simulink model "VehicleModel_Embedded"  (R2022a)
settings: Solver=FixedStepAuto  StartTime=0.0  StopTime=10.0  FixedStep=0.2  RelTol=1e-3
model workspace: external: MAT-File InitialValueFile.mat (data not in the file)
values from neighbouring files (symbols this model uses):
  DRIVER_EYES_OFF = Simulink.Parameter    [InitialValueFile.m]
  DRIVER_EYES_ON = Simulink.Parameter    [InitialValueFile.m]
  DRIVER_READINESS_HIGH = Simulink.Parameter    [InitialValueFile.m]
  DRIVER_READINESS_MEDIUM = Simulink.Parameter    [InitialValueFile.m]
  DRIVER_SEATED_ON = Simulink.Parameter    [InitialValueFile.m]
libraries: simulink x6
settings Model: Creator=HP  LastModifiedBy=HP
settings OptimizationCC: DefaultParameterBehavior=Inlined  EnhancedBackFolding=on  PassReuseOutputArgsAs=Individual arguments  ZeroExternalMemoryAtStartup=off  ZeroInternalMemoryAtStartup=off  OptimizeBlockOrder=speed  DifferentSizesBufferReuse=on  OptimizationCustomize=off  EfficientTunableParamExpr=on
settings DebuggingCC: ParameterTunabilityLossMsg=error
settings SFSimCC: MATLABDynamicMemAlloc=off
settings RTWCC: SystemTargetFile=ert.tlc  GenCodeOnly=on  TemplateMakefile=ert_default_tmf
settings CodeAppCC: ForceParamTrailComments=on  IgnoreCustomStorageClasses=off  OperatorAnnotations=on  SimulinkDataObjDesc=on  SFDataObjDesc=on  InsertBlockDesc=on
settings ERTTargetCC: TargetLangStandard=C99 (ISO)  GenerateSampleERTMain=on  InlinedParameterPlacement=NonHierarchical  ERTCustomFileTemplate=example_file_process.tlc

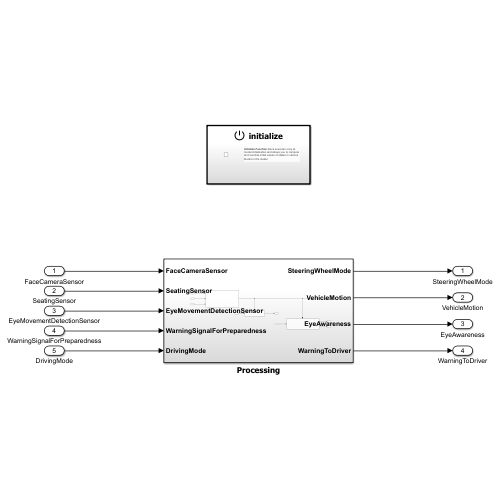
[thumbnail: Simulink's stored preview of the top-level diagram]
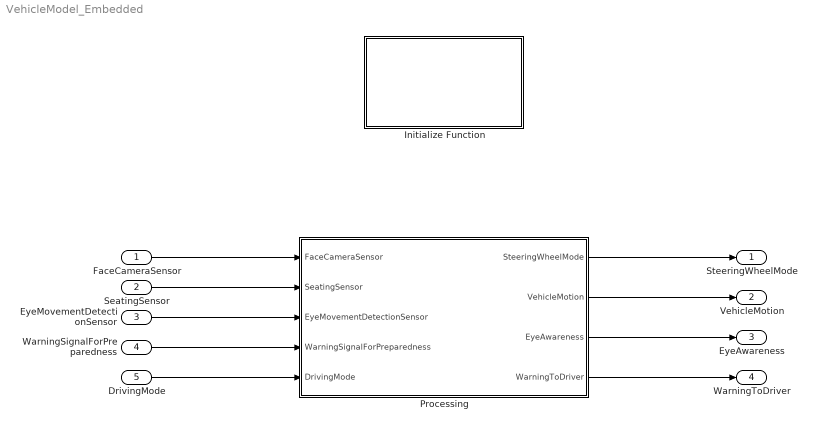
== system VehicleModel_Embedded ==
  FaceCameraSensor : Inport
  SeatingSensor : Inport  Port=2
  EyeMovementDetectionSensor : Inport  Port=3
  WarningSignalForPreparedness : Inport  Port=4
  DrivingMode : Inport  Port=5
  Initialize Function : Subsystem  TreatAsAtomicUnit=on
  Processing : Subsystem  SystemSampleTime=1
  SteeringWheelMode : Outport  VectorParamsAs1DForOutWhenUnconnected=off
  VehicleMotion : Outport  Port=2  VectorParamsAs1DForOutWhenUnconnected=off
  EyeAwareness : Outport  Port=3  VectorParamsAs1DForOutWhenUnconnected=off
  WarningToDriver : Outport  Port=4  VectorParamsAs1DForOutWhenUnconnected=off
  wires:
  Processing/4(WarningToDriver) -> WarningToDriver/1
  Processing/1(SteeringWheelMode) -> SteeringWheelMode/1
  EyeMovementDetectionSensor/1 -> Processing/3(EyeMovementDetectionSensor)
  DrivingMode/1 -> Processing/5(DrivingMode)
  FaceCameraSensor/1 -> Processing/1(FaceCameraSensor)
  SeatingSensor/1 -> Processing/2(SeatingSensor)
  WarningSignalForPreparedness/1 -> Processing/4(WarningSignalForPreparedness)
  Processing/2(VehicleMotion) -> VehicleMotion/1
  Processing/3(EyeAwareness) -> EyeAwareness/1

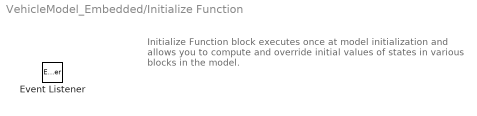
== system VehicleModel_Embedded/Initialize Function ==
  note: Initialize Function block executes once at model initialization and allows you to compute and override initial values of states in various blocks in the model.
  Event Listener : EventListener  DisableCoverage=on  EventName=reset

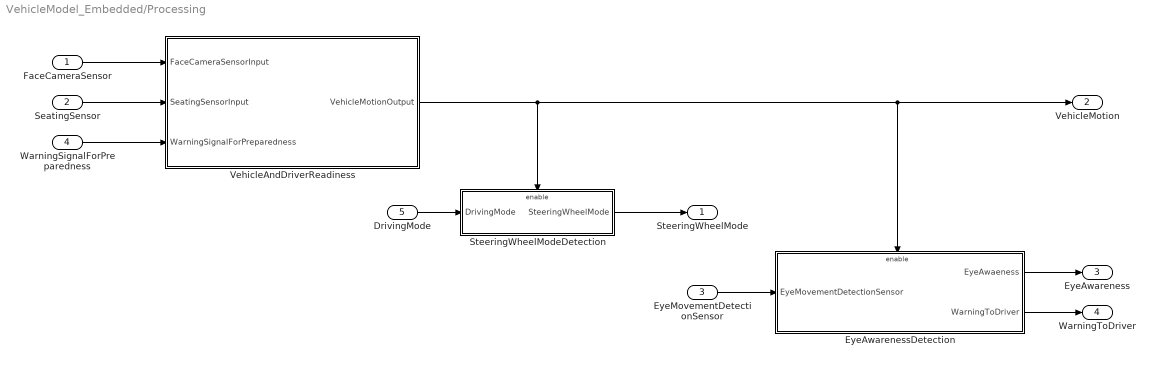
== system VehicleModel_Embedded/Processing ==
  FaceCameraSensor : Inport
  SeatingSensor : Inport  Port=2
  EyeMovementDetectionSensor : Inport  Port=3
  WarningSignalForPreparedness : Inport  Port=4
  DrivingMode : Inport  Port=5
  EyeAwarenessDetection : Subsystem
  SteeringWheelModeDetection : Subsystem
  VehicleAndDriverReadiness : Subsystem
  SteeringWheelMode : Outport  VectorParamsAs1DForOutWhenUnconnected=off
  VehicleMotion : Outport  Port=2  VectorParamsAs1DForOutWhenUnconnected=off
  EyeAwareness : Outport  Port=3
  WarningToDriver : Outport  Port=4
  wires:
  FaceCameraSensor/1 -> VehicleAndDriverReadiness/1(FaceCameraSensorInput)
  SeatingSensor/1 -> VehicleAndDriverReadiness/2(SeatingSensorInput)
  WarningSignalForPreparedness/1 -> VehicleAndDriverReadiness/3(WarningSignalForPreparedness)
  VehicleAndDriverReadiness/1(VehicleMotionOutput) -> VehicleMotion/1, EyeAwarenessDetection/Enable, SteeringWheelModeDetection/Enable
  EyeMovementDetectionSensor/1 -> EyeAwarenessDetection/1(EyeMovementDetectionSensor)
  SteeringWheelModeDetection/1(SteeringWheelMode) -> SteeringWheelMode/1
  EyeAwarenessDetection/1(EyeAwaeness) -> EyeAwareness/1
  DrivingMode/1 -> SteeringWheelModeDetection/1(DrivingMode)
  EyeAwarenessDetection/2(WarningToDriver) -> WarningToDriver/1

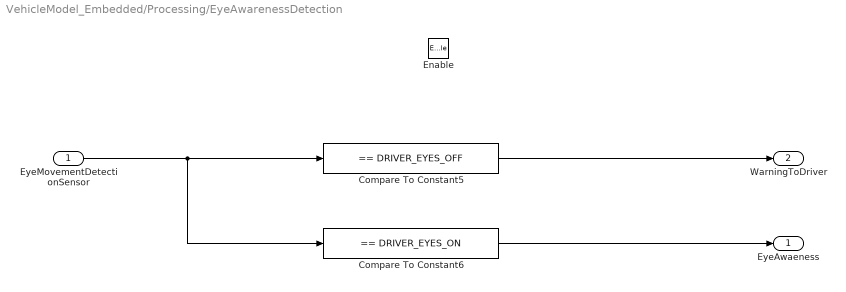
== system VehicleModel_Embedded/Processing/EyeAwarenessDetection ==
  EyeMovementDetectionSensor : Inport
  Enable : EnablePort
  Compare To Constant5 : simulink/Logic and Bit Operations/Compare To Constant  relop===  const=DRIVER_EYES_OFF  OutDataTypeStr=boolean
  Compare To Constant6 : simulink/Logic and Bit Operations/Compare To Constant  relop===  const=DRIVER_EYES_ON  OutDataTypeStr=boolean
  EyeAwaeness : Outport
  WarningToDriver : Outport  Port=2
  wires:
  Compare To Constant5/1 -> WarningToDriver/1
  Compare To Constant6/1 -> EyeAwaeness/1
  EyeMovementDetectionSensor/1 -> Compare To Constant6/1, Compare To Constant5/1

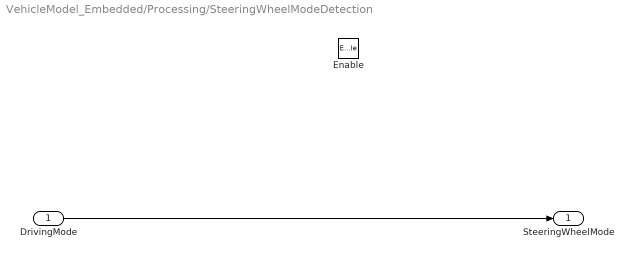
== system VehicleModel_Embedded/Processing/SteeringWheelModeDetection ==
  DrivingMode : Inport
  Enable : EnablePort
  SteeringWheelMode : Outport
  wires:
  DrivingMode/1 -> SteeringWheelMode/1

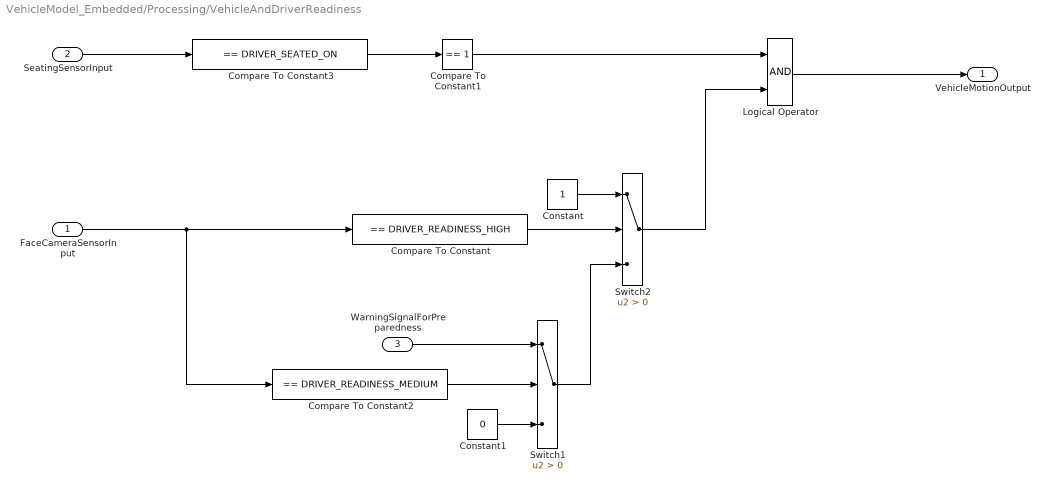
== system VehicleModel_Embedded/Processing/VehicleAndDriverReadiness ==
  FaceCameraSensorInput : Inport
  SeatingSensorInput : Inport  Port=2
  WarningSignalForPreparedness : Inport  Port=3
  Compare To Constant : simulink/Logic and Bit Operations/Compare To Constant  relop===  const=DRIVER_READINESS_HIGH  OutDataTypeStr=boolean
  Compare To Constant1 : simulink/Logic and Bit Operations/Compare To Constant  relop===  const=1  OutDataTypeStr=boolean
  Compare To Constant2 : simulink/Logic and Bit Operations/Compare To Constant  relop===  const=DRIVER_READINESS_MEDIUM  OutDataTypeStr=boolean
  Compare To Constant3 : simulink/Logic and Bit Operations/Compare To Constant  relop===  const=DRIVER_SEATED_ON  OutDataTypeStr=boolean
  Constant : Constant
  Constant1 : Constant  Value=0
  Logical Operator : Logic  AllPortsSameDT=off  OutDataTypeStr=boolean
  Switch1 : Switch  Criteria=u2 > Threshold  SaturateOnIntegerOverflow=off  InputSameDT=off
  Switch2 : Switch  Criteria=u2 > Threshold  SaturateOnIntegerOverflow=off  InputSameDT=off
  VehicleMotionOutput : Outport  VectorParamsAs1DForOutWhenUnconnected=off
  wires:
  Compare To Constant1/1 -> Logical Operator/1
  Switch1/1 -> Switch2/3
  Compare To Constant2/1 -> Switch1/2
  WarningSignalForPreparedness/1 -> Switch1/1
  Compare To Constant3/1 -> Compare To Constant1/1
  Compare To Constant/1 -> Switch2/2
  Constant/1 -> Switch2/1
  FaceCameraSensorInput/1 -> Compare To Constant/1, Compare To Constant2/1
  Constant1/1 -> Switch1/3
  SeatingSensorInput/1 -> Compare To Constant3/1
  Logical Operator/1 -> VehicleMotionOutput/1
  Switch2/1 -> Logical Operator/2
